simulink model "W5_Basic_Simulations"  (R2025b)
settings: Solver=VariableStepAuto  StartTime=0.0  StopTime=10.0  RelTol=1e-3
libraries: simulink x2
settings Model: Creator=MMD  LastModifiedBy=MMD

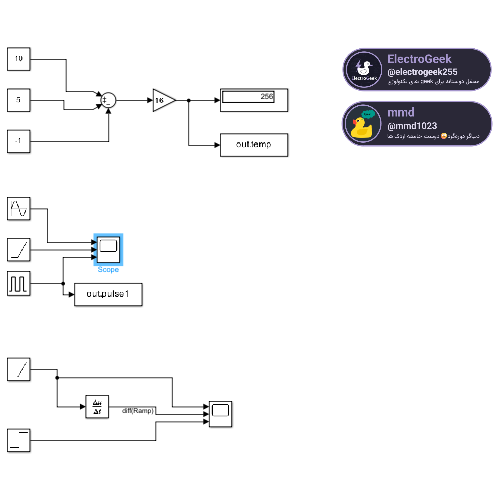
[thumbnail: Simulink's stored preview of the top-level diagram]
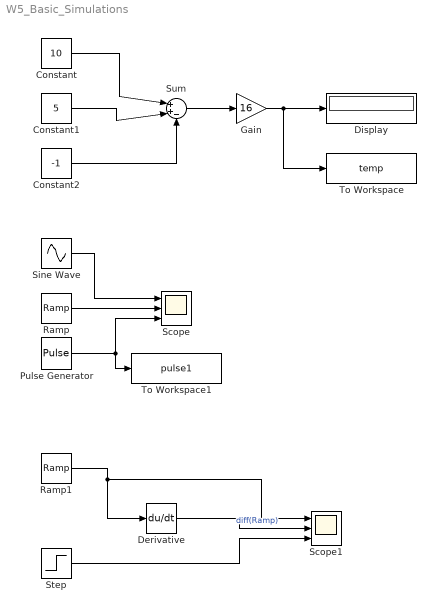
== system W5_Basic_Simulations ==
  Constant : Constant  Value=10
  Constant1 : Constant  Value=5
  Constant2 : Constant  Value=-1
  Derivative : Derivative
  Display : Display
  Gain : Gain  Gain=16
  Pulse Generator : DiscretePulseGenerator  PulseType=Time based  Amplitude=3.3  PulseWidth=50
  Ramp : simulink/Sources/Ramp  slope=1  start=2  InitialOutput=0
  Ramp1 : simulink/Sources/Ramp  slope=1  start=2  InitialOutput=0
  Scope : Scope  NumInputPorts=3
      settings: ActiveDisplayYMinimum=-2.1206851849403203  ActiveDisplayYMaximum=9.12452057610448
  Scope1 : Scope  NumInputPorts=3
      settings: ActiveDisplayYMinimum=-0.99999999999999978  ActiveDisplayYMaximum=9
  Sine Wave : Sin  SampleTime=0
  Step : Step  Time=2  SampleTime=0
  Sum : Sum  Inputs=|++-
  To Workspace : ToWorkspace  VariableName=temp  SaveFormat=Timeseries  SampleTime=-1
  To Workspace1 : ToWorkspace  VariableName=pulse1  SaveFormat=Timeseries  SampleTime=-1
  wires:
  Constant/1 -> Sum/1
  Constant1/1 -> Sum/2
  Constant2/1 -> Sum/3
  Sum/1 -> Gain/1
  Gain/1 -> To Workspace/1, Display/1
  Pulse Generator/1 -> To Workspace1/1, Scope/3
  Ramp/1 -> Scope/2
  Ramp1/1 -> Derivative/1, Scope1/1
  Derivative/1 -> Scope1/2  "diff(Ramp)"
  Step/1 -> Scope1/3
  Sine Wave/1 -> Scope/1
